simulink model "Derivative_Integral"  (R2020a)
settings: Solver=VariableStepAuto  StartTime=0.0  StopTime=10.0  RelTol=1e-3
settings Model: Creator=Mohammad  LastModifiedBy=Mohammad

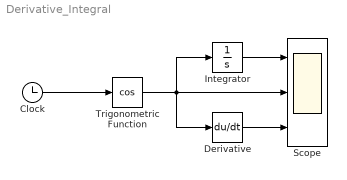
== system Derivative_Integral ==
  Clock : Clock
  Derivative : Derivative
  Integrator : Integrator
  Scope : Scope  NumInputPorts=3
  Trigonometric Function : Trigonometry  Operator=cos
  wires:
  Derivative/1 -> Scope/3
  Trigonometric Function/1 -> Integrator/1, Scope/2, Derivative/1
  Integrator/1 -> Scope/1
  Clock/1 -> Trigonometric Function/1
